simulink model "A2_PID"  (R2012b)
settings: Solver=ode45  StartTime=0.0  StopTime=500  RelTol=1e-3
PreLoadFcn:
  | Initialize
StopFcn:
  | A2_plot_and_save
undefined symbols (not defined in the file or in its folder): P, PlotTanks2
libraries: simulink x4, simulink_need_slupdate x2
settings Model: Creator=tsladeche  LastModifiedBy=John
settings DataIOCC: SignalLoggingSaveFormat=ModelDataLogs
settings DebuggingCC: FcnCallInpInsideContextMsg=UseLocalSettings  StrictBusMsg=Warning
settings GRTTargetCC: CombineOutputUpdateFcns=off  GRTInterface=on

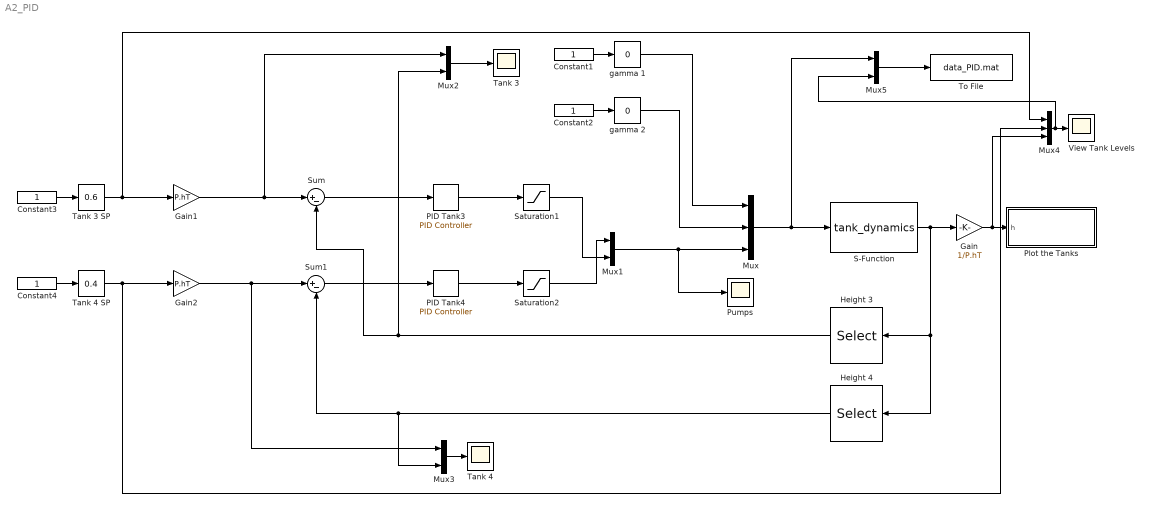
== system A2_PID ==
  Constant{1..4} (4 alike) : Constant
  Gain : Gain  Gain=1/P.hT
  Gain1 : Gain  Gain=P.hT
  Gain2 : Gain  Gain=P.hT
  Height 3 : Selector  InputPortWidth=4  IndexOptions=Index vector (dialog)  Indices=3  OutputSizes=1
  Height 4 : Selector  InputPortWidth=4  IndexOptions=Index vector (dialog)  Indices=4  OutputSizes=1
  Mux : Mux  Inputs=3
  Mux{1..3,5} (4 alike) : Mux  Inputs=2
  Mux4 : Mux  Inputs=3
  PID Tank3 : simulink_need_slupdate/PID Controller  P=.2  I=.001  D=0
  PID Tank4 : simulink_need_slupdate/PID Controller  P=.2  I=.001  D=0
  Plot the Tanks : Subsystem
  Pumps : Scope
      settings: TimeRange=200  YMin=0.05  YMax=1  SaveName=ScopeData3
  S-Function : S-Function  FunctionName=tank_dynamics  Parameters=P  EnableBusSupport=off
  Saturation1 : Saturate  UpperLimit=1  LowerLimit=.001
  Saturation2 : Saturate  UpperLimit=1  LowerLimit=.001
  Sum : Sum  Inputs=|+-
  Sum1 : Sum  Inputs=|+-
  Tank 3 : Scope
      settings: TimeRange=150  YMin=0  YMax=30
  Tank 3 SP : simulink/Math Operations/Slider Gain  low=0  gain=0.6  high=1
  Tank 4 : Scope
      settings: TimeRange=150  YMin=18.25  YMax=21.75  SaveName=ScopeData2
  Tank 4 SP : simulink/Math Operations/Slider Gain  low=0  gain=0.4  high=1
  To File : ToFile  Filename=data_PID.mat  MatrixName=tanks  SampleTime=1
  View Tank Levels : Scope
      settings: YMin=0.1  YMax=1.05  MaxDataPoints=50000
  gamma 1 : simulink/Math Operations/Slider Gain  low=0  gain=0  high=1
  gamma 2 : simulink/Math Operations/Slider Gain  low=0  gain=0  high=1
  wires:
  Constant2/1 -> gamma 2/1
  Constant1/1 -> gamma 1/1
  gamma 1/1 -> Mux/1
  gamma 2/1 -> Mux/2
  Gain/1 -> Mux4/3, Plot the Tanks/1(h)
  S-Function/1 -> Height 4/1, Height 3/1, Gain/1
  Mux/1 -> Mux5/1, S-Function/1
  Constant3/1 -> Tank 3 SP/1
  Constant4/1 -> Tank 4 SP/1
  Tank 4 SP/1 -> Mux4/2, Gain2/1
  Tank 3 SP/1 -> Mux4/1, Gain1/1
  Gain1/1 -> Sum/1, Mux2/1
  Gain2/1 -> Sum1/1, Mux3/1
  Sum/1 -> PID Tank3/1
  Sum1/1 -> PID Tank4/1
  Height 3/1 -> Sum/2, Mux2/2
  Height 4/1 -> Mux3/2, Sum1/2
  Mux1/1 -> Pumps/1, Mux/3
  PID Tank3/1 -> Saturation1/1
  PID Tank4/1 -> Saturation2/1
  Mux2/1 -> Tank 3/1
  Mux3/1 -> Tank 4/1
  Mux4/1 -> Mux5/2, View Tank Levels/1
  Mux5/1 -> To File/1
  Saturation1/1 -> Mux1/2
  Saturation2/1 -> Mux1/1

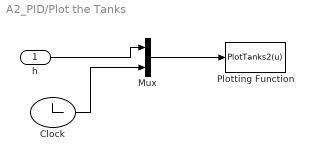
== system A2_PID/Plot the Tanks ==
  h : Inport
  Clock : Clock
  Mux : Mux  Inputs=2
  Plotting Function : MATLABFcn  MATLABFcn=PlotTanks2(u)  OutputDimensions=0  SampleTime=.05
  wires:
  Mux/1 -> Plotting Function/1
  Clock/1 -> Mux/2
  h/1 -> Mux/1
